simulink model "new_fin_opt_cont"  (Simulink 7.7)
settings: Solver=ode45  StartTime=0.0  StopTime=10.0  RelTol=1e-3
undefined symbols (not defined in the file or in its folder): fuzz_wght_2_corr
libraries: neural x1308
(part 29 of 29)

== system new_fin_opt_cont/loc_rod/net_loc_rod_3/Layer 3/Delays 1 ==
  "p{3}" : Inport  PortDimensions=50
      mask Display: e = 0.06;c1 = [120 230 180]/255;c2 = ([120 230 180]+0)/(256+128);c3 = ([120 230 180]+128)/(256+128);patch([0 1 1 0],[0 0 1 1],c1);patch([0 1 1 1-e 1-e 0+e],[0 0 1 1-e 0+e 0+e],c2);patch([0 0 1 1-e 0+e 0+e],[0 1 1 1-e 1-e 0+e],c3);plot([0 1 1 0 0],[0 0 1 1 0]);
  mux : Mux  Inputs=1
      mask Display: e = 0.06;c1 = [120 150 230]/255;c2 = ([120 150 230]+0)/383;c3 = ([120 150 230]+128)/383;patch([0 1 1 0],[0 0 1 1],c1);patch([0 1 1 1-e 1-e 0+e],[0 0 1 1-e 0+e 0+e],c2);patch([0 0 1 1-e 0+e 0+e],[0 1 1 1-e 1-e 0+e],c3);plot([0 1 1 0 0],[0 0 1 1 0]);disp('Mux')
  "pd{3,2}" : Outport
      mask Display: e = 0.06;c1 = [120 230 180]/255;c2 = ([120 230 180]+0)/(256+128);c3 = ([120 230 180]+128)/(256+128);patch([0 1 1 0],[0 0 1 1],c1);patch([0 1 1 1-e 1-e 0+e],[0 0 1 1-e 0+e 0+e],c2);patch([0 0 1 1-e 0+e 0+e],[0 1 1 1-e 1-e 0+e],c3);plot([0 1 1 0 0],[0 0 1 1 0]);
  wires:
  "p{3}"/1 -> mux/1
  mux/1 -> "pd{3,2}"/1

== system new_fin_opt_cont/loc_rod/net_loc_rod_3/Layer 3/LW{3,2} ==
  "ad{3,2}" : Inport  PortDimensions=50
      mask Display: e = 0.06;c1 = [120 230 180]/255;c2 = ([120 230 180]+0)/(256+128);c3 = ([120 230 180]+128)/(256+128);patch([0 1 1 0],[0 0 1 1],c1);patch([0 1 1 1-e 1-e 0+e],[0 0 1 1-e 0+e 0+e],c2);patch([0 0 1 1-e 0+e 0+e],[0 1 1 1-e 1-e 0+e],c3);plot([0 1 1 0 0],[0 0 1 1 0]);
  "IW{3,2}(1,:)'" : Constant  Value=[-0.053622316472408407;-0.84226494554242493;-0.011666555238415236;0.031159601043217352;-0.78268054928841213;-0.57151616164870489;1.4221727363549186;-0.10488946281125493;1.2411615794211213;0.43780555871349264;1.00493419279436;0.15002998915696672;1.3661578283373133;0.32486908955250487;-1.6329340060075963;-0.99013071211446091;-1.4892538432867246;0.26723088508392268;0.28734888528890729;0.58759079281789517;-0.1768652514762607;2.0048651876864887;0.56854832738280303;0.10563682831731072;-1.1861340597610985;-0.31187236193084056;-0.55652712678917171;-0.58570701720904939;-0.85769655120661814;-0.63504220012530976;-0.45945614747951691;-0.33497460021449971;0.44174526290521743;0.062041618499131916;0.68222669067813013;-1.0201721966018633;0.62059126174744772;0.95620224591382819;0.89174621526738795;-1.5292658096581986;-0.87351124103449762;0.1574652567038724;0.90406111130103139;0.70729979329683113;1.0917999447906963;0.85585506304082049;0.22171915966860506;0.075303211080594651;-0.96463296762836814;-1.4561106375539434]
      mask Display: e = 0.06;c1 = [120 150 230]/255;c2 = ([120 150 230]+0)/383;c3 = ([120 150 230]+128)/383;patch([0 1 1 0],[0 0 1 1],c1);patch([0 1 1 1-e 1-e 0+e],[0 0 1 1-e 0+e 0+e],c2);patch([0 0 1 1-e 0+e 0+e],[0 1 1 1-e 1-e 0+e],c3);plot([0 1 1 0 0],[0 0 1 1 0]);disp('weights');
  Mux : Mux  Inputs=1
      mask Display: e = 0.06;c1 = [120 150 230]/255;c2 = ([120 150 230]+0)/383;c3 = ([120 150 230]+128)/383;patch([0 1 1 0],[0 0 1 1],c1);patch([0 1 1 1-e 1-e 0+e],[0 0 1 1-e 0+e 0+e],c2);patch([0 0 1 1-e 0+e 0+e],[0 1 1 1-e 1-e 0+e],c3);plot([0 1 1 0 0],[0 0 1 1 0]);disp('Mux');
  dotprod1 : neural/Weight Functions/dotprod  SystemSampleTime=-1
  "lz{3,2}" : Outport
      mask Display: e = 0.06;c1 = [120 230 180]/255;c2 = ([120 230 180]+0)/(256+128);c3 = ([120 230 180]+128)/(256+128);patch([0 1 1 0],[0 0 1 1],c1);patch([0 1 1 1-e 1-e 0+e],[0 0 1 1-e 0+e 0+e],c2);patch([0 0 1 1-e 0+e 0+e],[0 1 1 1-e 1-e 0+e],c3);plot([0 1 1 0 0],[0 0 1 1 0]);
  wires:
  "IW{3,2}(1,:)'"/1 -> dotprod1/1
  "ad{3,2}"/1 -> dotprod1/2
  dotprod1/1 -> Mux/1
  Mux/1 -> "lz{3,2}"/1

== matlab function Subsystem1/MATLAB Function ==
  data: t input double; y output double; fuz_wgt input double
function y = fcn(t,fuz_wgt)
if t<=100
    y=fuz_wgt(4,1);
elseif t<=200
    y=fuz_wgt(4,2);
elseif t<=300
    y=fuz_wgt(4,3);
elseif t<=400
    y=fuz_wgt(4,4);
elseif t<=500
    y=fuz_wgt(4,5);
else
    y=fuz_wgt(4,6);
end
end

== matlab function Subsystem2/MATLAB Function ==
  data: t input double; y output double; fuz_wgt input double
function y = fcn(t,fuz_wgt)
if t<=100
    y=fuz_wgt(4,1);
elseif t<=200
    y=fuz_wgt(4,2);
elseif t<=300
    y=fuz_wgt(4,3);
elseif t<=400
    y=fuz_wgt(4,4);
elseif t<=500
    y=fuz_wgt(4,5);
else
    y=fuz_wgt(4,6);
end
end

== matlab function Subsystem/MATLAB Function ==
  data: t input double; y output double; fuz_wgt input double
function y = fcn(t,fuz_wgt)
if t<=100
    y=fuz_wgt(4,1);
elseif t<=200
    y=fuz_wgt(4,2);
elseif t<=300
    y=fuz_wgt(4,3);
elseif t<=400
    y=fuz_wgt(4,4);
elseif t<=500
    y=fuz_wgt(4,5);
else
    y=fuz_wgt(4,6);
end
end

== matlab function Subsystem3/MATLAB Function ==
  data: t input double; y output double; fuz_wgt input double
function y = fcn(t,fuz_wgt)
if t<=100
    y=fuz_wgt(4,1);
elseif t<=200
    y=fuz_wgt(4,2);
elseif t<=300
    y=fuz_wgt(4,3);
elseif t<=400
    y=fuz_wgt(4,4);
elseif t<=500
    y=fuz_wgt(4,5);
else
    y=fuz_wgt(4,6);
end
end
